simulink model "DrivingDistanceD3D4"  (R2018b)
settings: Solver=VariableStepAuto  StartTime=0.0  StopTime=1000  RelTol=1e-3
settings Model: Creator=gregoryseibert  LastModifiedBy=gregoryseibert

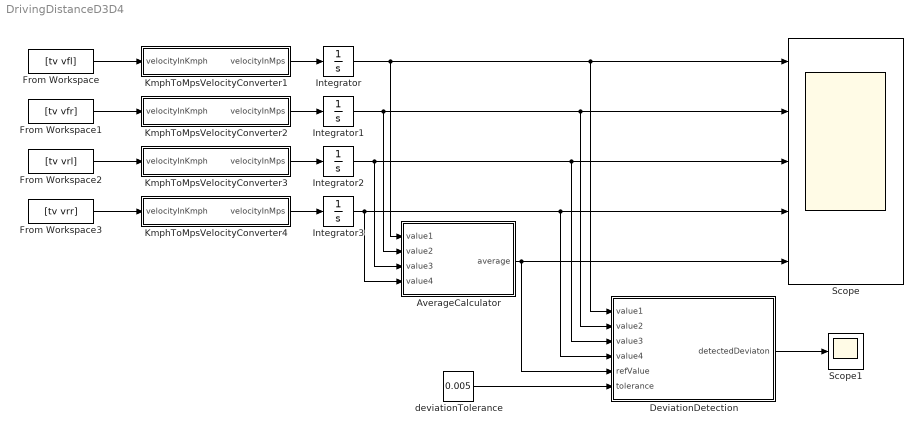
== system DrivingDistanceD3D4 ==
  AverageCalculator : Subsystem
  DeviationDetection : Subsystem
  From Workspace : FromWorkspace  VariableName=[tv vfl]  SampleTime=0
  From Workspace1 : FromWorkspace  VariableName=[tv vfr]  SampleTime=0
  From Workspace2 : FromWorkspace  VariableName=[tv vrl]  SampleTime=0
  From Workspace3 : FromWorkspace  VariableName=[tv vrr]  SampleTime=0
  Integrator{,1..3} (4 alike) : Integrator
  KmphToMpsVelocityConverter1 : Subsystem
  KmphToMpsVelocityConverter2 : Subsystem
  KmphToMpsVelocityConverter3 : Subsystem
  KmphToMpsVelocityConverter4 : Subsystem
  Scope : Scope  NumInputPorts=5
  Scope1 : Scope
  deviationTolerance : Constant  Value=0.005
  wires:
  Integrator/1 -> AverageCalculator/1(value1), DeviationDetection/1(value1), Scope/1
  Integrator1/1 -> AverageCalculator/2(value2), DeviationDetection/2(value2), Scope/2
  Integrator2/1 -> AverageCalculator/3(value3), DeviationDetection/3(value3), Scope/3
  Integrator3/1 -> AverageCalculator/4(value4), DeviationDetection/4(value4), Scope/4
  deviationTolerance/1 -> DeviationDetection/6(tolerance)
  DeviationDetection/1(detectedDeviaton) -> Scope1/1
  AverageCalculator/1(average) -> DeviationDetection/5(refValue), Scope/5
  From Workspace/1 -> KmphToMpsVelocityConverter1/1(velocityInKmph)
  KmphToMpsVelocityConverter1/1(velocityInMps) -> Integrator/1
  KmphToMpsVelocityConverter4/1(velocityInMps) -> Integrator3/1
  From Workspace1/1 -> KmphToMpsVelocityConverter2/1(velocityInKmph)
  From Workspace2/1 -> KmphToMpsVelocityConverter3/1(velocityInKmph)
  From Workspace3/1 -> KmphToMpsVelocityConverter4/1(velocityInKmph)
  KmphToMpsVelocityConverter3/1(velocityInMps) -> Integrator2/1
  KmphToMpsVelocityConverter2/1(velocityInMps) -> Integrator1/1

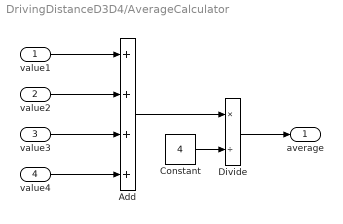
== system DrivingDistanceD3D4/AverageCalculator ==
  value1 : Inport
  value2 : Inport  Port=2
  value3 : Inport  Port=3
  value4 : Inport  Port=4
  Add : Sum  Inputs=++++
  Constant : Constant  Value=4
  Divide : Product  Inputs=*/
  average : Outport
  wires:
  value4/1 -> Add/4
  value3/1 -> Add/3
  Divide/1 -> average/1
  value2/1 -> Add/2
  value1/1 -> Add/1
  Constant/1 -> Divide/2
  Add/1 -> Divide/1

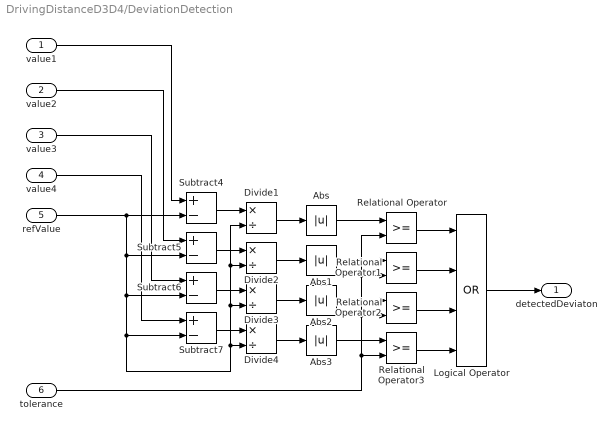
== system DrivingDistanceD3D4/DeviationDetection ==
  value1 : Inport
  value2 : Inport  Port=2
  value3 : Inport  Port=3
  value4 : Inport  Port=4
  refValue : Inport  Port=5
  tolerance : Inport  Port=6
  Abs{,1..3} (4 alike) : Abs
  Divide{1..4} (4 alike) : Product  Inputs=*/
  Logical Operator : Logic  Operator=OR  Inputs=4  AllPortsSameDT=off  OutDataTypeStr=boolean
  Relational Operator{,1..3} (4 alike) : RelationalOperator  OutDataTypeStr=boolean  RndMeth=Simplest
  Subtract{4..7} (4 alike) : Sum  Inputs=+-
  detectedDeviaton : Outport
  wires:
  value1/1 -> Subtract4/1
  Subtract6/1 -> Divide3/1
  Subtract4/1 -> Divide1/1
  Subtract5/1 -> Divide2/1
  Abs1/1 -> Relational Operator1/1
  Logical Operator/1 -> detectedDeviaton/1
  Abs3/1 -> Relational Operator3/1
  Relational Operator/1 -> Logical Operator/1
  Relational Operator1/1 -> Logical Operator/2
  Relational Operator2/1 -> Logical Operator/3
  Divide4/1 -> Abs3/1
  value3/1 -> Subtract6/1
  Divide1/1 -> Abs/1
  value2/1 -> Subtract5/1
  tolerance/1 -> Relational Operator/2, Relational Operator1/2, Relational Operator2/2, Relational Operator3/2
  value4/1 -> Subtract7/1
  Subtract7/1 -> Divide4/1
  Abs/1 -> Relational Operator/1
  Relational Operator3/1 -> Logical Operator/4
  Divide3/1 -> Abs2/1
  Abs2/1 -> Relational Operator2/1
  Divide2/1 -> Abs1/1
  refValue/1 -> Subtract7/2, Divide4/2, Divide3/2, Divide2/2, Divide1/2, Subtract6/2, Subtract5/2, Subtract4/2

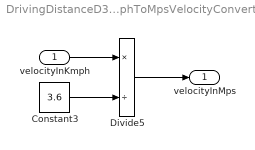
== system DrivingDistanceD3D4/KmphToMpsVelocityConverter1 ==
  velocityInKmph : Inport
  Constant3 : Constant  Value=3.6
  Divide5 : Product  Inputs=*/
  velocityInMps : Outport
  wires:
  Divide5/1 -> velocityInMps/1
  velocityInKmph/1 -> Divide5/1
  Constant3/1 -> Divide5/2

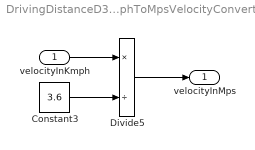
== system DrivingDistanceD3D4/KmphToMpsVelocityConverter2 ==
  velocityInKmph : Inport
  Constant3 : Constant  Value=3.6
  Divide5 : Product  Inputs=*/
  velocityInMps : Outport
  wires:
  Divide5/1 -> velocityInMps/1
  velocityInKmph/1 -> Divide5/1
  Constant3/1 -> Divide5/2

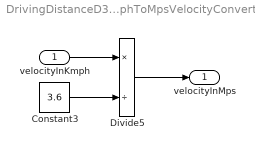
== system DrivingDistanceD3D4/KmphToMpsVelocityConverter3 ==
  velocityInKmph : Inport
  Constant3 : Constant  Value=3.6
  Divide5 : Product  Inputs=*/
  velocityInMps : Outport
  wires:
  Divide5/1 -> velocityInMps/1
  velocityInKmph/1 -> Divide5/1
  Constant3/1 -> Divide5/2

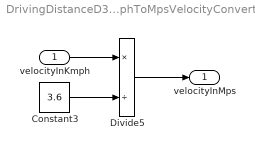
== system DrivingDistanceD3D4/KmphToMpsVelocityConverter4 ==
  velocityInKmph : Inport
  Constant3 : Constant  Value=3.6
  Divide5 : Product  Inputs=*/
  velocityInMps : Outport
  wires:
  Divide5/1 -> velocityInMps/1
  velocityInKmph/1 -> Divide5/1
  Constant3/1 -> Divide5/2
